simulink model "clik_z_inverse"  (R2022b)
settings: Solver=ode1  StartTime=0.0  StopTime=4  FixedStep=0.001  RelTol=1e-3
undefined symbols (not defined in the file or in its folder): DiscIntNeverNeededParam, q0, Tc
settings Model: Creator=Xp  LastModifiedBy=CHINMAY PRASHANTH
settings SolverCC: AlgebraicLoopSolver=TrustRegion
settings DataIOCC: LimitDataPoints=on  SaveFormat=Array  SignalLoggingSaveFormat=ModelDataLogs  ReturnWorkspaceOutputs=off
settings OptimizationCC: ExpressionDepthLimit=2147483647  InitFltsAndDblsToZero=on  LifeSpan=inf
settings DebuggingCC: SaveWithParameterizedLinksMsg=none  UnderspecifiedInitializationDetection=Classic  MergeDetectMultiDrivingBlocksExec=none  SolverPrmCheckMsg=warning  MultiTaskDSMMsg=warning  MultiTaskCondExecSysMsg=none  FcnCallInpInsideContextMsg=warning  UnconnectedInputMsg=warning  UnconnectedOutputMsg=warning  UnconnectedLineMsg=warning  StateNameClashWarn=warning  SFUnexpectedBacktrackingDiag=warning  SFNoUnconditionalDefaultTransitionDiag=warning  SFExecutionAtInitializationDiag=none  SFMachineParentedDataDiag=warning  ArithmeticOperatorsInVariantConditions=warning
settings HardwareCC: ProdBitPerPointer=32  ProdBitPerSizeT=32  ProdBitPerPtrDiffT=32  ProdLargestAtomicFloat=None  ProdIntDivRoundTo=Undefined  ProdEndianess=Unspecified  ProdWordSize=32  ProdHWDeviceType=32-bit Generic
settings ModelReferenceCC: EnableRefExpFcnMdlSchedulingChecks=on  PropagateSignalLabelsOutOfModel=off
settings SFSimCC: CustomCodeUndefinedFunction=UseInterfaceOnly
settings RTWCC: DLArmComputeVersion=19.05
settings CodeAppCC: StateflowObjectComments=on
settings GRTTargetCC: TargetLangStandard=C89/C90 (ANSI)  CombineOutputUpdateFcns=off  GRTInterface=on
settings ConfigComp: CovMetricSettings=dw  CovSaveCumulativeToWorkspaceVar=on  CovSaveSingleToWorkspaceVar=on

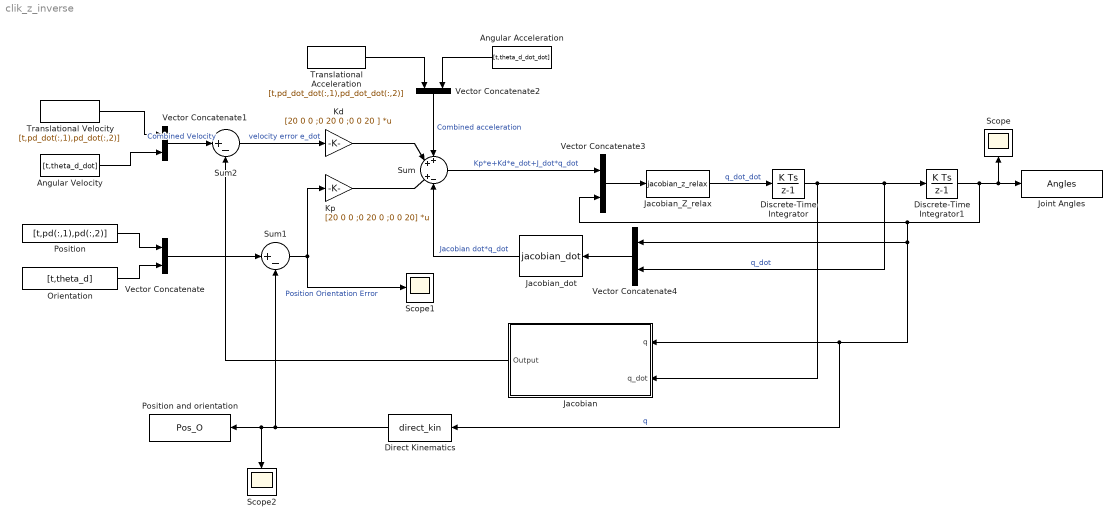
== system clik_z_inverse ==
  Angular Acceleration : FromWorkspace  VariableName=[t,theta_d_dot_dot]
  Angular Velocity : FromWorkspace  VariableName=[t,theta_d_dot]
  Direct Kinematics : MATLABFcn  MATLABFcn=direct_kin  OutputDimensions=3
  Discrete-Time Integrator : DiscreteIntegrator  InitialCondition=[0;0;0;0]  SampleTime=Tc  ICPrevOutput=DiscIntNeverNeededParam  ICPrevScaledInput=DiscIntNeverNeededParam
  Discrete-Time Integrator1 : DiscreteIntegrator  InitialCondition=q0  SampleTime=Tc  LimitOutput=on  UpperSaturationLimit=[inf;inf;1;inf]  LowerSaturationLimit=[-inf; -inf; 0.25; -inf]  ICPrevOutput=DiscIntNeverNeededParam  ICPrevScaledInput=DiscIntNeverNeededParam
  "Jacobian " : MATLAB Function  TreatAsAtomicUnit=on
  Jacobian_Z_relax : MATLABFcn  MATLABFcn=jacobian_z_relax  OutputDimensions=4
  Jacobian_dot : MATLABFcn  MATLABFcn=jacobian_dot  OutputDimensions=3
  Joint Angles : ToWorkspace  VariableName=Angles  SampleTime=-1
      settings: Save2DSignal=2-D array (concatenate along first dimension)
  Kd : Gain  Gain=[20 0 0 ;0 20 0 ;0 0 20 ]  Multiplication=Matrix(K*u)
  Kp : Gain  Gain=[20 0 0 ;0 20 0 ;0 0 20]  Multiplication=Matrix(K*u)
  Orientation : FromWorkspace  VariableName=[t,theta_d]
  Position : FromWorkspace  VariableName=[t,pd(:,1),pd(:,2)]
  Position and orientation : ToWorkspace  VariableName=Pos_O  SampleTime=-1
  Scope : Scope
  Scope1 : Scope
  Scope2 : Scope
  Sum : Sum  Inputs=++|+-
  Sum1 : Sum  Inputs=|+-
  Sum2 : Sum  Inputs=|+-
  "Translational Acceleration " : FromWorkspace  VariableName=[t,pd_dot_dot(:,1),pd_dot_dot(:,2)]
  Translational Velocity : FromWorkspace  VariableName=[t,pd_dot(:,1),pd_dot(:,2)]
  Vector Concatenate{,1..4} (5 alike) : Concatenate
  wires:
  Kd/1 -> Sum/2
  Orientation/1 -> Vector Concatenate/2
  Vector Concatenate1/1 -> Sum2/1  "Combined Velocity"
  Discrete-Time Integrator1/1 -> Joint Angles/1, Scope/1, Vector Concatenate3/2, Direct Kinematics/1, "Jacobian "/1(q), Vector Concatenate4/1  "q"
  Angular Acceleration/1 -> Vector Concatenate2/2
  Sum/1 -> Vector Concatenate3/1  "Kp*e+Kd*e_dot+J_dot*q_dot"
  Angular Velocity/1 -> Vector Concatenate1/2
  "Jacobian "/1(Output) -> Sum2/2
  Vector Concatenate/1 -> Sum1/1
  Vector Concatenate3/1 -> Jacobian_Z_relax/1
  Jacobian_Z_relax/1 -> Discrete-Time Integrator/1  "q_dot_dot"
  Translational Velocity/1 -> Vector Concatenate1/1
  Sum1/1 -> Scope1/1, Kp/1  "Position Orientation Error"
  Vector Concatenate4/1 -> Jacobian_dot/1
  Sum2/1 -> Kd/1  "velocity error e_dot"
  Kp/1 -> Sum/3
  "Translational Acceleration "/1 -> Vector Concatenate2/1
  Vector Concatenate2/1 -> Sum/1  "Combined acceleration"
  Jacobian_dot/1 -> Sum/4  "Jacobian dot*q_dot"
  Direct Kinematics/1 -> Scope2/1, Position and orientation/1, Sum1/2
  Discrete-Time Integrator/1 -> Vector Concatenate4/2, Discrete-Time Integrator1/1, "Jacobian "/2(q_dot)  "q_dot"
  Position/1 -> Vector Concatenate/1

== matlab function clik_z_inverse/Jacobian  ==
  data: q input; Output output; q_dot input
function Output= fcn(q,q_dot)

    Theta1=q(1);
    
    Theta2=q(2);

    a1=0.5;
    
    a2=0.5;
    
    Jacobian=[- a2*sin(Theta1 + Theta2) - a1*sin(Theta1), -a2*sin(Theta1 + Theta2), 0, 0; a2*cos(Theta1 + Theta2) + a1*cos(Theta1), a2*cos(Theta1 + Theta2), 0,0; 1, 1, 0, 1];
    
    Output=Jacobian*q_dot;

end
